simulink library "Storage_Type_4"  (Simulink 8.2)
settings: Solver=ode45  StartTime=0.0  StopTime=10.0  RelTol=1e-3
libraries: carnot x7
settings Model: Creator=lena.frank  LastModifiedBy=drhf

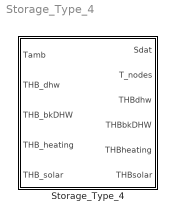
== system Storage_Type_4 ==
  Storage_Type_4 : Subsystem  mask(Multiport Storage){uloss=0.74, ubot=1.37, utop=0.74, cond=0.62, t0=[10:5:55], volume=0.75, dia=0.79, pos=standing cylinder, nconnect=4, nodes=50, mpoints=50}
      mask prompts: uloss "Heat loss coefficient cylinder wall in W/(m²K)"; ubot "Heat loss coefficient bottom in W/(m²K)"; utop "Heat loss coefficient top cover in W/(m²K)"; cond "Effective (wall and fluid) vertical conductivity in W/(m*K)"; t0 "Initial temperature (vector or scalar) in °C"; volume "Volume in m³"; dia "Diameter in m"; pos "Position"; nconnect "Number of connections"; nodes "Number of nodes"; mpoints "Number of measurement points"
      mask help:
      | The volmue of the cylindrical storage is divided in a number "nodes" of horizontal slices (1xN-node model). For each node the energy balance equation is solved.
      | Look under mask to set the ports types and properties.
      mask init:
      | [standing, dh, height, mpts, tini] ...
      |     = CarnotCallbacks_StorageTypeN(pos, volume, dia, nodes, mpoints, t0);
      mask Help: web(fullfile(path_carnot('help'),'Storage_Type_N.html'),'-helpbrowser')
      mask TypeOptions pos: lying cylinder | standing cylinder
      mask Display: plot(5,10,85,110,[36,36,40,50,54,54,50,40,36],[90,50,45,45,50,90,93,93,90],[36,51,40,51,36],[50,50,68,85,85],[36,51,44,51,36],[54,54,56,58,58])

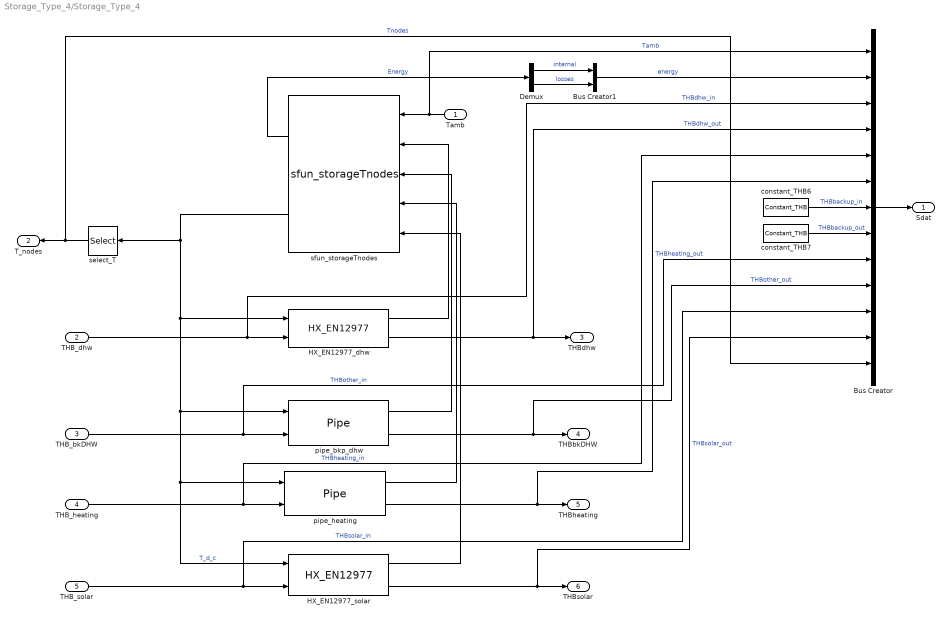
== system Storage_Type_4/Storage_Type_4 ==
  Tamb : Inport
  THB_dhw : Inport  Port=2
  THB_bkDHW : Inport  Port=3
  THB_heating : Inport  Port=4
  THB_solar : Inport  Port=5
  Bus Creator : BusCreator  Inputs=13
  Bus Creator1 : BusCreator  Inputs=2
  Demux : Demux  Outputs=2
  HX_EN12977_dhw : carnot/Storage/Thermal/Storage_Ports/HX_EN12977  h_in=0.02  h_out=0.95  ua0=642.2  uam=0.369  uat=0.684  dplin=100  dpqua=100  nodes=nodes  hgt=height  dia=dia
  HX_EN12977_solar : carnot/Storage/Thermal/Storage_Ports/HX_EN12977  h_in=0.45  h_out=0  ua0=678.6  uam=0.411  uat=0.287  dplin=100  dpqua=100  nodes=nodes  hgt=height  dia=dia
  constant_THB6 : carnot/Source/Simple/Constant_THB  t=20  mdot=0  p=1e5  mID=No Pressure Drop  fluid=Water  mix=0  dia=0.02  hgt=0
  constant_THB7 : carnot/Source/Simple/Constant_THB  t=20  mdot=0  p=1e5  mID=No Pressure Drop  fluid=Water  mix=0  dia=0.02  hgt=0
  pipe_bkp_dhw : carnot/Storage/Thermal/Storage_Ports/Pipe  h_in=1  h_out=0.54  dplin=10  dpqua=10  nodes=nodes  hgt=height  dia=dia
  pipe_heating : carnot/Storage/Thermal/Storage_Ports/Pipe  h_in=0.45  h_out=0.54  dplin=10  dpqua=10  nodes=nodes  hgt=height  dia=dia
  select_T : Selector  InputPortWidth=nodes  IndexOptions=Index vector (dialog)  Indices=mpts  OutputSizes=1
  sfun_storageTnodes : carnot/Basic/Thermal_Models/sfun_storageTnodes  dia=dia  volume=volume  standing=standing  uloss=uloss  ubot=utop  utop=ubot  cond=cond  tini=tini  nodes=nodes  nconnect=nconnect
  Sdat : Outport
  T_nodes : Outport  Port=2
  THBdhw : Outport  Port=3
  THBbkDHW : Outport  Port=4
  THBheating : Outport  Port=5
  THBsolar : Outport  Port=6
  wires:
  constant_THB7/1 -> Bus Creator/8  "THBbackup_out"
  constant_THB6/1 -> Bus Creator/7  "THBbackup_in"
  pipe_heating/2 -> Bus Creator/6, THBheating/1  "THBheating_out"
  HX_EN12977_solar/1 -> sfun_storageTnodes/5
  pipe_heating/1 -> sfun_storageTnodes/4
  THB_heating/1 -> Bus Creator/5, pipe_heating/2  "THBheating_in"
  Tamb/1 -> sfun_storageTnodes/1, Bus Creator/1  "Tamb"
  THB_dhw/1 -> HX_EN12977_dhw/2, Bus Creator/3  "THBdhw_in"
  HX_EN12977_dhw/2 -> THBdhw/1, Bus Creator/4  "THBdhw_out"
  HX_EN12977_dhw/1 -> sfun_storageTnodes/2
  select_T/1 -> T_nodes/1, Bus Creator/13  "Tnodes"
  sfun_storageTnodes/1 -> Demux/1  "Energy"
  sfun_storageTnodes/2 -> select_T/1, HX_EN12977_dhw/1, pipe_heating/1, HX_EN12977_solar/1, pipe_bkp_dhw/1  "T_d_c"
  Bus Creator/1 -> Sdat/1
  THB_bkDHW/1 -> Bus Creator/9, pipe_bkp_dhw/2  "THBother_in"
  pipe_bkp_dhw/2 -> Bus Creator/10, THBbkDHW/1  "THBother_out"
  pipe_bkp_dhw/1 -> sfun_storageTnodes/3
  Demux/1 -> Bus Creator1/1  "internal"
  Demux/2 -> Bus Creator1/2  "losses"
  Bus Creator1/1 -> Bus Creator/2  "energy"
  THB_solar/1 -> HX_EN12977_solar/2, Bus Creator/11  "THBsolar_in"
  HX_EN12977_solar/2 -> THBsolar/1, Bus Creator/12  "THBsolar_out"
